simulink model "SubSystem4Layers4Blocks"  (Simulink 7.6)
settings: Solver=ode45  StartTime=0.0  StopTime=10.0  RelTol=1e-3
settings Model: Creator=DominikC  LastModifiedBy=DominikC
settings DebuggingCC: FcnCallInpInsideContextMsg=Enable All

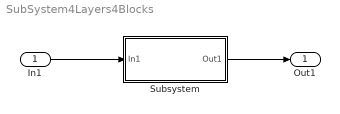
== system SubSystem4Layers4Blocks ==
  In1 : Inport
  Subsystem : Subsystem
  Out1 : Outport
  wires:
  In1/1 -> Subsystem/1(In1)
  Subsystem/1(Out1) -> Out1/1

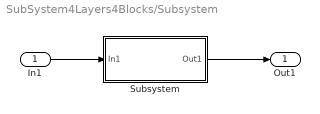
== system SubSystem4Layers4Blocks/Subsystem ==
  In1 : Inport
  Subsystem : Subsystem
  Out1 : Outport
  wires:
  In1/1 -> Subsystem/1(In1)
  Subsystem/1(Out1) -> Out1/1

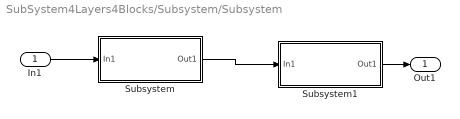
== system SubSystem4Layers4Blocks/Subsystem/Subsystem ==
  In1 : Inport
  Subsystem : Subsystem
  Subsystem1 : Subsystem
  Out1 : Outport
  wires:
  In1/1 -> Subsystem/1(In1)
  Subsystem1/1(Out1) -> Out1/1
  Subsystem/1(Out1) -> Subsystem1/1(In1)

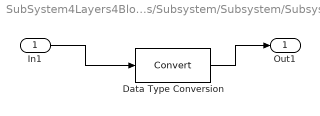
== system SubSystem4Layers4Blocks/Subsystem/Subsystem/Subsystem ==
  In1 : Inport
  Data Type Conversion : DataTypeConversion
  Out1 : Outport
  wires:
  In1/1 -> Data Type Conversion/1
  Data Type Conversion/1 -> Out1/1

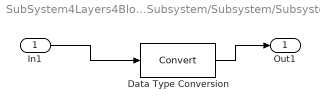
== system SubSystem4Layers4Blocks/Subsystem/Subsystem/Subsystem1 ==
  In1 : Inport
  Data Type Conversion : DataTypeConversion
  Out1 : Outport
  wires:
  In1/1 -> Data Type Conversion/1
  Data Type Conversion/1 -> Out1/1
